simulink model "task_2"  (Simulink 7.6)
settings: Solver=ode45  StartTime=0.0  StopTime=1  RelTol=1e-3
settings Model: Creator=Admin  LastModifiedBy=Admin

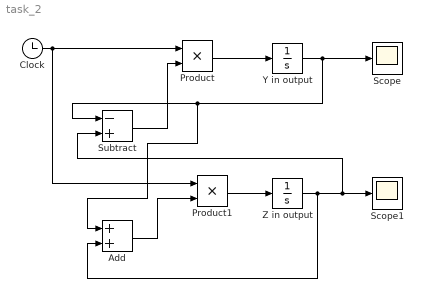
== system task_2 ==
  Add : Sum
  Clock : Clock
      settings: Decimation=10
  Product : Product  RndMeth=Zero
  Product1 : Product  RndMeth=Zero
  Scope : Scope
  Scope1 : Scope
  Subtract : Sum  Inputs=-+
  Y in output : Integrator  InitialCondition=1
  Z in output : Integrator  InitialCondition=1
  wires:
  Clock/1 -> Product/1, Product1/1
  Z in output/1 -> Add/2, Subtract/2, Scope1/1
  Y in output/1 -> Subtract/1, Add/1, Scope/1
  Product/1 -> Y in output/1
  Subtract/1 -> Product/2
  Product1/1 -> Z in output/1
  Add/1 -> Product1/2
